simulink library "simulink"  (R2016b)
settings: Solver=ode45  StartTime=0.0  StopTime=10.0  RelTol=1e-3
PostLoadFcn:
  | setsysloc_simulink(bdroot)
undefined symbols (not defined in the file): DiscIntNeverNeededParam, docblock, getdatatypespecs, NumBits1, NumBits2, sfunxy, sigbuilder_block, slcm, SlDemoSign, Slope1, Slope2
libraries: simulink x37, sl_helperblocks x2, eml_lib x1
(part 6 of 6)

== system simulink/Sources/Chirp Signal ==
  note: freqSlope = deltaFreq/targetTime;
      | instantaneousFreq(t) = freqSlope*t + initialFreq;
      | intantaneousPhase(t) = integral(instFreq) = ...
      |       0.5*freqSlope*t^2 + initialFreq*t;
      | outputSignal(t) = sin(instantaneousPhase(t));
  Clock1 : Clock
      settings: DisableCoverage=on
  Gain : Gain  DisableCoverage=on  Gain=0.5  OutDataTypeStr=Inherit: Same as input  ParamDataTypeStr=Inherit: Same as input
  Output : Trigonometry
  Product : Product  DisableCoverage=on  Inputs=*/  SaturateOnIntegerOverflow=on  InputSameDT=on  OutDataTypeStr=Inherit: Same as first input
  Product1 : Product  DisableCoverage=on  SaturateOnIntegerOverflow=on  InputSameDT=on  OutDataTypeStr=Inherit: Same as first input
  Product2 : Product  DisableCoverage=on  SaturateOnIntegerOverflow=on  InputSameDT=on  OutDataTypeStr=Inherit: Same as first input
  Sum : Sum  DisableCoverage=on  Inputs=|++  SaturateOnIntegerOverflow=on  InputSameDT=on  OutDataTypeStr=Inherit: Same as first input
  deltaFreq : Constant  DisableCoverage=on  Value=2*pi*(f2-f1)
  initialFreq : Constant  DisableCoverage=on  Value=2*pi*f1
  targetTime : Constant  DisableCoverage=on  Value=T
  y : Outport
  wires:
  deltaFreq/1 -> Product/1
  targetTime/1 -> Product/2
  Product/1 -> Gain/1
  Clock1/1 -> Product1/1, Product2/1
  Gain/1 -> Product1/2
  Product1/1 -> Sum/1
  initialFreq/1 -> Sum/2
  Sum/1 -> Product2/2
  Product2/1 -> Output/1
  Output/1 -> y/1

== system simulink/Sources/Counter Free-Running ==
  FixPt Data Type Propagation : simulink/Signal Attributes/Data Type Propagation  PropDataTypeMode=Specify via dialog  PropDataType=uint(NumBits)  IfRefDouble=double  IfRefSingle=single  IsSigned=IsSigned1 or IsSigned2  NumBitsBase=max([NumBits1 NumBits2])  NumBitsMult=1  NumBitsAdd=0  NumBitsAllowFinal=1:128  PropScalingMode=Specify via dialog  PropScaling=1  ValuesUsedBestPrec=[5 -7]  SlopeBase=min([Slope1 Slope2])  SlopeMult=1  SlopeAdd=0  BiasBase=Bias1  BiasMult=1  BiasAdd=0
  Force to be scalar : SignalSpecification  DisableCoverage=on  Dimensions=1
  Increment Real World : simulink/Additional Math & Discrete/Additional Math: Increment - Decrement/Increment Real World  DisableCoverage=on
  Output : UnitDelay  InitialCondition=0.0  SampleTime=tsamp
  Wrap To Zero : simulink/Discontinuities/Wrap To Zero  DisableCoverage=on  Threshold=(2^(NumBits))-1
  y : Outport
  wires:
  Force to be scalar/1 -> Increment Real World/1
  Wrap To Zero/1 -> Output/1, FixPt Data Type Propagation/1, FixPt Data Type Propagation/3, FixPt Data Type Propagation/2
  Increment Real World/1 -> Wrap To Zero/1
  Output/1 -> Force to be scalar/1, y/1

== system simulink/Sources/Counter Limited ==
  Data Type Propagation : simulink/Signal Attributes/Data Type Propagation  PropDataTypeMode=Specify via dialog  PropDataType=uint(nbits)  IfRefDouble=double  IfRefSingle=single  IsSigned=IsSigned1 or IsSigned2  NumBitsBase=max([NumBits1 NumBits2])  NumBitsMult=1  NumBitsAdd=0  NumBitsAllowFinal=1:128  PropScalingMode=Specify via dialog  PropScaling=1  ValuesUsedBestPrec=[5 -7]  SlopeBase=min([Slope1 Slope2])  SlopeMult=1  SlopeAdd=0  BiasBase=Bias1  BiasMult=1  BiasAdd=0
  Force to be scalar : SignalSpecification  DisableCoverage=on  Dimensions=1
  Increment Real World : simulink/Additional Math & Discrete/Additional Math: Increment - Decrement/Increment Real World  DisableCoverage=on
  Output : UnitDelay  InitialCondition=0.0  SampleTime=tsamp
  Wrap To Zero : simulink/Discontinuities/Wrap To Zero  DisableCoverage=on  Threshold=uplimit
  y : Outport
  wires:
  Force to be scalar/1 -> Increment Real World/1
  Increment Real World/1 -> Wrap To Zero/1
  Output/1 -> Force to be scalar/1, y/1
  Wrap To Zero/1 -> Data Type Propagation/3, Data Type Propagation/2, Data Type Propagation/1, Output/1

== system simulink/Sources/Enumerated Constant ==
  Constant : Constant  DialogController=Simulink.DDGSource  Value=SlDemoSign.Positive  OutDataTypeStr=Enum: SlDemoSign  LockScale=on
  Out : Outport
  wires:
  Constant/1 -> Out/1

== system simulink/Sources/Ramp ==
  Clock : Clock
      settings: DisableCoverage=on
  Constant : Constant  DisableCoverage=on  Value=start  OutDataTypeStr=Inherit: Inherit via back propagation
  Constant1 : Constant  DisableCoverage=on  Value=X0  OutDataTypeStr=Inherit: Inherit via back propagation
  Output : Sum  Inputs=|++  SaturateOnIntegerOverflow=on  InputSameDT=on  OutDataTypeStr=Inherit: Same as first input
  Product : Product  DisableCoverage=on  SaturateOnIntegerOverflow=on  InputSameDT=on  OutDataTypeStr=Inherit: Same as first input
  Step : Step  DisableCoverage=on  Time=start  After=slope  SampleTime=0
  Sum : Sum  DisableCoverage=on  Inputs=|+-  SaturateOnIntegerOverflow=on  InputSameDT=on  OutDataTypeStr=Inherit: Same as first input
  Out1 : Outport
  wires:
  Step/1 -> Product/1
  Product/1 -> Output/1
  Constant1/1 -> Output/2
  Output/1 -> Out1/1
  Sum/1 -> Product/2
  Constant/1 -> Sum/2
  Clock/1 -> Sum/1

== system simulink/Sources/Repeating Sequence ==
  Clock : Clock
      settings: DisableCoverage=on
  Constant : Constant  DisableCoverage=on  Value=period
  Look-Up Table1 : Lookup_n-D  DisableCoverage=on  NumberOfTableDimensions=1  BreakpointsForDimension1=rep_seq_t - min(rep_seq_t)  BreakpointsForDimension3=[5, 7]  Table=rep_seq_y  InternalRulePriority=Speed  SaturateOnIntegerOverflow=on  InputSameDT=on
  Math Function : Math  DisableCoverage=on  Operator=rem  SaturateOnIntegerOverflow=on
  Output : SignalConversion  OverrideOpt=off
  Sum : Sum  DisableCoverage=on  Inputs=+-  SaturateOnIntegerOverflow=on  InputSameDT=on  OutDataTypeStr=Inherit: Same as first input
  startTime : S-Function  DisableCoverage=on  FunctionName=sfun_tstart  SFunctionDeploymentMode=off  EnableBusSupport=off
  Out1 : Outport
  wires:
  Math Function/1 -> Look-Up Table1/1
  Sum/1 -> Math Function/1
  Clock/1 -> Sum/1
  startTime/1 -> Sum/2
  Look-Up Table1/1 -> Output/1
  Output/1 -> Out1/1
  Constant/1 -> Math Function/2

== system simulink/Sources/Repeating Sequence Interpolated ==
  Data Type Propagation : simulink/Signal Attributes/Data Type Propagation  PropDataType=fixdt(1, 16)  IfRefDouble=double  IfRefSingle=single  IsSigned=IsSigned2  NumBitsBase=NumBits2  NumBitsMult=1  NumBitsAdd=0  NumBitsAllowFinal=1:128  PropScaling=2^-10  ValuesUsedBestPrec=[5 -7]  SlopeBase=Slope2  SlopeMult=1  SlopeAdd=0  BiasBase=Bias2  BiasMult=1  BiasAdd=0
  Data Type Conversion : DataTypeConversion  DisableCoverage=on
  Force to be scalar : SignalSpecification  DisableCoverage=on  Dimensions=1
  LimitedCounter : simulink/Sources/Counter Limited  uplimit=nn  tsamp=tsamp
  Lookup : Lookup_n-D  DisableCoverage=on  NumberOfTableDimensions=1  BreakpointsForDimension1=TimeValues  BreakpointsForDimension3=[5, 7]  Table=OutValues  ExtrapMethod=Clip  OutMin=OutMin  OutMax=OutMax  OutDataTypeStr=OutDataTypeStr  InputSameDT=on
  Output : SignalConversion  OverrideOpt=off
  Sample Time Math : SampleTimeMath  DisableCoverage=on  TsampMathOp=*  TsampMathImp=Offline Scaling Adjustment
  y : Outport  OutMin=OutMin  OutMax=OutMax
  wires:
  Output/1 -> y/1
  Lookup/1 -> Output/1, Data Type Propagation/1
  Force to be scalar/1 -> Data Type Conversion/1, Data Type Propagation/2
  LimitedCounter/1 -> Force to be scalar/1
  Sample Time Math/1 -> Lookup/1
  Data Type Conversion/1 -> Sample Time Math/1, Data Type Propagation/3

== system simulink/Sources/Repeating Sequence Stair ==
  Force to be scalar : SignalSpecification  DisableCoverage=on  Dimensions=1
  LimitedCounter : simulink/Sources/Counter Limited  uplimit=nn  tsamp=tsamp
  Out : SignalConversion  OverrideOpt=off
  Output : MultiPortSwitch  DisableCoverage=on  DataPortOrder=Zero-based contiguous  Inputs=1  zeroidx=on  OutMin=OutMin  OutMax=OutMax  SampleTime=tsamp
  Vector : Constant  DisableCoverage=on  Value=OutValues  OutMin=OutMin  OutMax=OutMax  OutDataTypeStr=OutDataTypeStr
  y : Outport  OutMin=OutMin  OutMax=OutMax
  wires:
  Force to be scalar/1 -> Output/1
  Vector/1 -> Output/2
  LimitedCounter/1 -> Force to be scalar/1
  Output/1 -> Out/1
  Out/1 -> y/1

== system simulink/Sources/Signal Builder ==
  Demux : Demux  Tag=STV Demux  Outputs=1
  FromWs : FromWorkspace  Tag=STV FromWs  VariableName=tuvar  SampleTime=0
      SigBuilderData=|
      | common.afterFinalStr = 'Extrapolate'
      | common.sampleTime = 0
      | dataSet.timeRange = [0 10]
      | dataSet.name = 'Group 1'
      | sbobj.Groups.Name = 'Group 1'
      | sbobj.Groups.Signals.Name = 'Signal 1'
      | sbobj.Groups.Signals.XData = [0 4 4 6 6 10]
      | sbobj.Groups.Signals.YData = [0 0 1 1 0 0]
  Signal 1 : Outport  Tag=STV Outport
  wires:
  FromWs/1 -> Demux/1
  Demux/1 -> Signal 1/1

== system simulink/Sources/Waveform Generator ==
  Converter : DataTypeConversion  OutMin=OutMin  OutMax=OutMax  OutDataTypeStr=double
  MultiportSwitch : MultiPortSwitch  Inputs=1
  MultiportSwitch_e3df3653d217406 : Ground  DisableCoverage=on
  Switch : Constant  DisableCoverage=on  Value=SelectedSignal
  Out1 : Outport
  wires:
  Switch/1 -> MultiportSwitch/1
  Converter/1 -> Out1/1
  MultiportSwitch/1 -> Converter/1
  MultiportSwitch_e3df3653d217406/1 -> MultiportSwitch/2

== system simulink/User-Defined Functions/Initialize Function ==
  Constant : Constant  DisableCoverage=on  Value=0
  Event Listener : EventListener  EventType=Initialize  EventName=reset
  State Writer : StateWriter
  wires:
  Constant/1 -> State Writer/1

== system simulink/User-Defined Functions/S-Function Examples ==
  Gain : Gain  SaturateOnIntegerOverflow=on  OutDataTypeStr=Inherit: Same as input  ParamDataTypeStr=Inherit: Same as input

== system simulink/User-Defined Functions/Simulink Function ==
  f : TriggerPort  TriggerType=function-call  IsSimulinkFunction=on  FunctionName=f  VariantControl=Variant
  u : ArgIn  DisableCoverage=on  ArgumentName=u
  y : ArgOut  DisableCoverage=on  ArgumentName=y
  wires:
  u/1 -> y/1

== system simulink/User-Defined Functions/Terminate Function ==
  Event Listener : EventListener  EventType=Terminate  EventName=reset
  State Reader : StateReader
  Terminator : Terminator
  wires:
  State Reader/1 -> Terminator/1

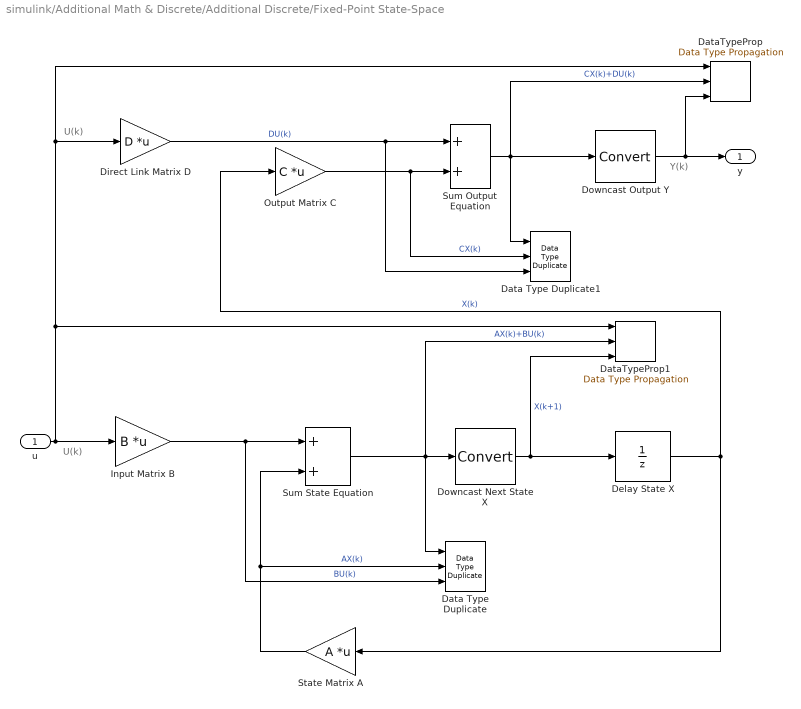
== system simulink/Additional Math & Discrete/Additional Discrete/Fixed-Point State-Space ==
  note: U(k)
  note: U(k)
  note: Y(k)
  u : Inport
  Data Type Duplicate : DataTypeDuplicate  DisableCoverage=on  NumInputPorts=3
  Data Type Duplicate1 : DataTypeDuplicate  DisableCoverage=on  NumInputPorts=3
  DataTypeProp : simulink/Signal Attributes/Data Type Propagation  PropDataType=fixdt(1, 16)  IfRefDouble=double  IfRefSingle=single  IsSigned=IsSigned1 or IsSigned2  NumBitsBase=NumBits1  NumBitsMult=1  NumBitsAdd=0  NumBitsAllowFinal=1:128  PropScaling=2^-10  ValuesUsedBestPrec=[5 -7]  SlopeBase=PosRange2  SlopeMult=1  SlopeAdd=0  BiasBase=Bias2  BiasMult=1  BiasAdd=0
  DataTypeProp1 : simulink/Signal Attributes/Data Type Propagation  PropDataType=fixdt(1, 16)  IfRefDouble=double  IfRefSingle=single  IsSigned=IsSigned1 or IsSigned2  NumBitsBase=NumBits1  NumBitsMult=1  NumBitsAdd=0  NumBitsAllowFinal=1:128  PropScaling=2^-10  ValuesUsedBestPrec=[5 -7]  SlopeBase=PosRange2  SlopeMult=1  SlopeAdd=0  BiasBase=Bias2  BiasMult=1  BiasAdd=0
  Delay State X : UnitDelay  Description=Store in Global RAM  DisableCoverage=on  InitialCondition=X0  SampleTime=-1
      settings: AttributesFormatString=%<Description>
  Direct Link Matrix D : Gain  Description=Multiply in CPU  DisableCoverage=on  Gain=D  Multiplication=Matrix(K*u) (u vector)  OutDataTypeStr=Inherit: Inherit via back propagation
      settings: AttributesFormatString=%<Description>
  Downcast Next State X : DataTypeConversion  Description=|  DisableCoverage=on
      | Reduce from CPU Size
      |  to Global RAM Size
      settings: AttributesFormatString=%<Description>
  Downcast Output Y : DataTypeConversion  Description=|
      | Reduce from CPU Size
      |  to Global RAM Size
      settings: AttributesFormatString=%<Description>
  Input Matrix B : Gain  Description=Multiply in CPU  DisableCoverage=on  Gain=B  Multiplication=Matrix(K*u) (u vector)  OutDataTypeStr=Inherit: Inherit via back propagation
      settings: AttributesFormatString=%<Description>
  Output Matrix C : Gain  Description=Multiply in CPU  DisableCoverage=on  Gain=C  Multiplication=Matrix(K*u) (u vector)  OutDataTypeStr=Inherit: Inherit via back propagation
      settings: AttributesFormatString=%<Description>
  State Matrix A : Gain  Description=Multiply in CPU  DisableCoverage=on  Gain=A  Multiplication=Matrix(K*u) (u vector)  OutDataTypeStr=Inherit: Inherit via back propagation
      settings: AttributesFormatString=%<Description>
  Sum Output Equation : Sum  Description=Add in CPU  DisableCoverage=on  OutDataTypeStr=slDataTypeAndScale(('InternalDataType'),('OutputEqScaling'))
      settings: AttributesFormatString=%<Description>
  Sum State Equation : Sum  Description=Add in CPU  DisableCoverage=on  OutDataTypeStr=slDataTypeAndScale(('InternalDataType'),('StateEqScaling'))
      settings: AttributesFormatString=%<Description>
  y : Outport  InitialOutput=0
  wires:
  Direct Link Matrix D/1 -> Data Type Duplicate1/3, Sum Output Equation/1  "DU(k)"
  Output Matrix C/1 -> Data Type Duplicate1/2, Sum Output Equation/2  "CX(k)"
  Sum Output Equation/1 -> DataTypeProp/2, Data Type Duplicate1/1, Downcast Output Y/1  "CX(k)+DU(k)"
  Downcast Output Y/1 -> DataTypeProp/3, y/1
  Delay State X/1 -> Output Matrix C/1, State Matrix A/1  "X(k)"
  Downcast Next State X/1 -> DataTypeProp1/3, Delay State X/1  "X(k+1)"
  Sum State Equation/1 -> DataTypeProp1/2, Data Type Duplicate/1, Downcast Next State X/1  "AX(k)+BU(k)"
  Input Matrix B/1 -> Data Type Duplicate/3, Sum State Equation/1  "BU(k)"
  u/1 -> DataTypeProp1/1, DataTypeProp/1, Direct Link Matrix D/1, Input Matrix B/1
  State Matrix A/1 -> Data Type Duplicate/2, Sum State Equation/2  "AX(k)"

== system simulink/Additional Math & Discrete/Additional Discrete/Transfer Fcn Direct Form II ==
  u : Inport
  DataTypeProp : simulink/Signal Attributes/Data Type Propagation  PropDataType=fixdt(1, 16)  IfRefDouble=double  IfRefSingle=single  IsSigned=IsSigned1 or IsSigned2  NumBitsBase=max([NumBits1 NumBits2])  NumBitsMult=1  NumBitsAdd=0  NumBitsAllowFinal=1:128  PropScaling=2^-10  ValuesUsedBestPrec=[5 -7]  SlopeBase=min([Slope1 Slope2])  SlopeMult=OutputSlopeMult  SlopeAdd=0  BiasBase=Bias1  BiasMult=0  BiasAdd=0
  DataTypeProp1 : simulink/Signal Attributes/Data Type Propagation  PropDataType=fixdt(1, 16)  IfRefDouble=double  IfRefSingle=single  IsSigned=IsSigned1 or IsSigned2  NumBitsBase=max([NumBits1 NumBits2])  NumBitsMult=1  NumBitsAdd=0  NumBitsAllowFinal=1:128  PropScaling=2^-10  ValuesUsedBestPrec=[5 -7]  SlopeBase=min([Slope1 Slope2])  SlopeMult=OutputSlopeMult2  SlopeAdd=0  BiasBase=Bias1  BiasMult=0  BiasAdd=0
  DenCoef : Gain  DisableCoverage=on  Gain=DenCoefVec  Multiplication=Matrix(K*u) (u vector)
      settings: AttributesFormatString=|
      | Data Type and Scaling Inherited
      | with goal of NO Quantization Noise
      | Possible Overflow or Saturation
  Downcast : DataTypeConversion  Description=|  LockScale=on
      | Reduce from CPU Size
      |  to Global RAM Size
      settings: AttributesFormatString=%<Description>
  Downcast1 : DataTypeConversion  Description=|  DisableCoverage=on  LockScale=on
      | Reduce from CPU Size
      |  to Global RAM Size
      settings: AttributesFormatString=%<Description>
  Mux : Mux  Inputs=2
  NumCoef : Gain  DisableCoverage=on  Gain=NumCoefVec  Multiplication=Matrix(K*u) (u vector)
      settings: AttributesFormatString=|
      | Data Type and Scaling Inherited
      | with goal of NO Quantization Noise
      | Possible Overflow or Saturation
  Sum : Sum  Tag=S16 2^-10  DisableCoverage=on  Inputs=+-  LockScale=on
      settings: AttributesFormatString=|
      | Data Type and Scaling Inherited
      | with goal of NO Quantization Noise
      | Possible Overflow or Saturation
  Tapped Delay : simulink/Discrete/Tapped Delay  vinit=vinit  samptime=-1  NumDelays=-1  DelayOrder=Newest  includeCurrent=off
      settings: AttributesFormatString=|
      | Number of Taps
      | Inherited via Back Propagation
  y : Outport
  wires:
  Sum/1 -> Downcast1/1
  DenCoef/1 -> Sum/2
  u/1 -> DataTypeProp1/1, DataTypeProp1/2, DataTypeProp/2, DataTypeProp/1, Sum/1
  NumCoef/1 -> Downcast/1
  Tapped Delay/1 -> DenCoef/1, Mux/2
  Downcast1/1 -> DataTypeProp1/3, Mux/1, Tapped Delay/1
  Mux/1 -> NumCoef/1
  Downcast/1 -> y/1, DataTypeProp/3

== system simulink/Additional Math & Discrete/Additional Discrete/Transfer Fcn Direct Form II Time Varying ==
  u : Inport
  Num : Inport  Port=2
  Den No Lead : Inport  Port=3
  DataTypeProp : simulink/Signal Attributes/Data Type Propagation  PropDataType=fixdt(1, 16)  IfRefDouble=double  IfRefSingle=single  IsSigned=IsSigned1  NumBitsBase=NumBits1  NumBitsMult=1  NumBitsAdd=0  NumBitsAllowFinal=1:128  PropScaling=2^-10  ValuesUsedBestPrec=[5 -7]  SlopeBase=Slope1  SlopeMult=1  SlopeAdd=0  BiasBase=Bias1  BiasMult=1  BiasAdd=0
  DataTypeProp1 : simulink/Signal Attributes/Data Type Propagation  PropDataType=fixdt(1, 16)  IfRefDouble=double  IfRefSingle=single  IsSigned=IsSigned1  NumBitsBase=NumBits1  NumBitsMult=1  NumBitsAdd=0  NumBitsAllowFinal=1:128  PropScaling=2^-10  ValuesUsedBestPrec=[5 -7]  SlopeBase=Slope1  SlopeMult=2  SlopeAdd=0  BiasBase=Bias1  BiasMult=1  BiasAdd=0
  Dot1 : DotProduct  DisableCoverage=on  OutDataTypeStr=Inherit: Inherit via internal rule
      settings: AttributesFormatString=|
      | Data Type and Scaling Inherited
      | with goal of NO Quantization Noise
      | Possible Overflow or Saturation
  Dot2 : DotProduct  DisableCoverage=on  OutDataTypeStr=Inherit: Inherit via internal rule
      settings: AttributesFormatString=|
      | Data Type and Scaling Inherited
      | with goal of NO Quantization Noise
      | Possible Overflow or Saturation
  Downcast : DataTypeConversion  Description=|  LockScale=on
      | Reduce from CPU Size
      |  to Global RAM Size
      settings: AttributesFormatString=%<Description>
  Downcast1 : DataTypeConversion  Description=|  DisableCoverage=on  LockScale=on
      | Reduce from CPU Size
      |  to Global RAM Size
      settings: AttributesFormatString=%<Description>
  Mux : Mux  Inputs=2
  Sum : Sum  Tag=S16 2^-10  DisableCoverage=on  Inputs=+-  LockScale=on
      settings: AttributesFormatString=|
      | Data Type and Scaling Inherited
      | with goal of NO Quantization Noise
      | Possible Overflow or Saturation
  Tapped Delay : simulink/Discrete/Tapped Delay  vinit=vinit  samptime=-1  NumDelays=-1  DelayOrder=Newest  includeCurrent=off
      settings: AttributesFormatString=|
      | Number of Taps
      | Inherited via Back Propagation
  y : Outport
  wires:
  Den No Lead/1 -> Dot1/2
  Num/1 -> Dot2/2
  Downcast/1 -> DataTypeProp/3, y/1
  Mux/1 -> Dot2/1
  Downcast1/1 -> DataTypeProp1/3, Tapped Delay/1, Mux/1
  Tapped Delay/1 -> Dot1/1, Mux/2
  Dot2/1 -> Downcast/1
  u/1 -> Sum/1, DataTypeProp1/2, DataTypeProp1/1, DataTypeProp/2, DataTypeProp/1
  Dot1/1 -> Sum/2
  Sum/1 -> Downcast1/1

== system simulink/Additional Math & Discrete/Additional Math: Increment - Decrement/Decrement Real World ==
  u : Inport
  FixPt Constant : Constant  DisableCoverage=on  OutDataTypeStr=Inherit: Inherit via back propagation
  FixPt Data Type Duplicate : DataTypeDuplicate  DisableCoverage=on  NumInputPorts=3
  FixPt Sum1 : Sum  Inputs=+-  OutDataTypeStr=Inherit: Inherit via back propagation  InputSameDT=on  LockScale=on
  y : Outport
  wires:
  FixPt Sum1/1 -> y/1, FixPt Data Type Duplicate/1
  FixPt Constant/1 -> FixPt Sum1/2, FixPt Data Type Duplicate/3
  u/1 -> FixPt Sum1/1, FixPt Data Type Duplicate/2

== system simulink/Additional Math & Discrete/Additional Math: Increment - Decrement/Decrement Stored Integer ==
  u : Inport
  FixPt Constant : Constant  DisableCoverage=on  OutDataTypeStr=Inherit: Inherit via back propagation
  FixPt Data Type Duplicate : DataTypeDuplicate  DisableCoverage=on  NumInputPorts=3
  FixPt Data Type Propagation : simulink/Signal Attributes/Data Type Propagation  PropDataType=fixdt(1, 16)  IfRefDouble=double  IfRefSingle=single  IsSigned=IsSigned1  NumBitsBase=NumBits1  NumBitsMult=1  NumBitsAdd=0  NumBitsAllowFinal=1:128  PropScaling=2^-10  ValuesUsedBestPrec=[5 -7]  SlopeBase=Slope1  SlopeMult=0  SlopeAdd=1  BiasBase=Bias1  BiasMult=0  BiasAdd=0
  FixPt Gateway In : DataTypeConversion  DisableCoverage=on  ConvertRealWorld=Stored Integer (SI)
  FixPt Sum1 : Sum  Inputs=+-  OutDataTypeStr=Inherit: Inherit via back propagation  InputSameDT=on  LockScale=on
  y : Outport
  wires:
  u/1 -> FixPt Data Type Duplicate/2, FixPt Sum1/1
  FixPt Constant/1 -> FixPt Gateway In/1, FixPt Data Type Propagation/3
  FixPt Sum1/1 -> FixPt Data Type Duplicate/1, y/1
  FixPt Gateway In/1 -> FixPt Data Type Duplicate/3, FixPt Sum1/2, FixPt Data Type Propagation/1, FixPt Data Type Propagation/2

== system simulink/Additional Math & Discrete/Additional Math: Increment - Decrement/Decrement To Zero ==
  u : Inport
  FixPt Constant : Constant  DisableCoverage=on  OutDataTypeStr=Inherit: Inherit via back propagation
  FixPt Data Type Duplicate : DataTypeDuplicate  DisableCoverage=on  NumInputPorts=5
  FixPt Relational Operator3 : RelationalOperator  DisableCoverage=on  Operator=>  OutDataTypeStr=boolean  ZeroCross=off  RndMeth=Nearest
  FixPt Sum1 : Sum  DisableCoverage=on  Inputs=+-  OutDataTypeStr=Inherit: Inherit via back propagation  LockScale=on
  FixPt Switch4 : Switch  Criteria=u2 ~= 0  Threshold=1  OutDataTypeStr=Inherit: Inherit via back propagation  ZeroCross=off
  Ground1 : Ground  DisableCoverage=on
  y : Outport
  wires:
  FixPt Switch4/1 -> FixPt Data Type Duplicate/1, y/1
  Ground1/1 -> FixPt Data Type Duplicate/2, FixPt Switch4/3
  FixPt Relational Operator3/1 -> FixPt Switch4/2
  u/1 -> FixPt Relational Operator3/1, FixPt Data Type Duplicate/4, FixPt Sum1/1
  FixPt Constant/1 -> FixPt Relational Operator3/2, FixPt Data Type Duplicate/5, FixPt Sum1/2
  FixPt Sum1/1 -> FixPt Switch4/1, FixPt Data Type Duplicate/3

== system simulink/Additional Math & Discrete/Additional Math: Increment - Decrement/Decrement Time To Zero ==
  u : Inport
  FixPt Data Type Duplicate : DataTypeDuplicate  DisableCoverage=on  NumInputPorts=5
  FixPt Relational Operator3 : RelationalOperator  DisableCoverage=on  Operator=>  OutDataTypeStr=boolean  ZeroCross=off  RndMeth=Nearest
  FixPt Sample Time Math : SampleTimeMath  DisableCoverage=on  TsampMathOp=Ts Only  OutDataTypeStr=Inherit: Inherit via back propagation
  FixPt Sum1 : Sum  DisableCoverage=on  Inputs=+-  OutDataTypeStr=Inherit: Inherit via back propagation  LockScale=on
  FixPt Switch4 : Switch  Criteria=u2 ~= 0  Threshold=1  OutDataTypeStr=Inherit: Inherit via back propagation  ZeroCross=off
  Ground1 : Ground  DisableCoverage=on
  y : Outport
  wires:
  FixPt Switch4/1 -> FixPt Data Type Duplicate/1, y/1
  Ground1/1 -> FixPt Data Type Duplicate/2, FixPt Switch4/3
  FixPt Relational Operator3/1 -> FixPt Switch4/2
  u/1 -> FixPt Relational Operator3/1, FixPt Data Type Duplicate/4, FixPt Sum1/1, FixPt Sample Time Math/1
  FixPt Sample Time Math/1 -> FixPt Relational Operator3/2, FixPt Data Type Duplicate/5, FixPt Sum1/2
  FixPt Sum1/1 -> FixPt Switch4/1, FixPt Data Type Duplicate/3

== system simulink/Additional Math & Discrete/Additional Math: Increment - Decrement/Increment Real World ==
  u : Inport
  FixPt Constant : Constant  DisableCoverage=on  OutDataTypeStr=Inherit: Inherit via back propagation
  FixPt Data Type Duplicate : DataTypeDuplicate  DisableCoverage=on  NumInputPorts=3
  FixPt Sum1 : Sum  OutDataTypeStr=Inherit: Inherit via back propagation  InputSameDT=on  LockScale=on
  y : Outport
  wires:
  u/1 -> FixPt Data Type Duplicate/2, FixPt Sum1/1
  FixPt Constant/1 -> FixPt Data Type Duplicate/3, FixPt Sum1/2
  FixPt Sum1/1 -> FixPt Data Type Duplicate/1, y/1

== system simulink/Additional Math & Discrete/Additional Math: Increment - Decrement/Increment Stored Integer ==
  u : Inport
  FixPt Constant : Constant  DisableCoverage=on  OutDataTypeStr=Inherit: Inherit via back propagation
  FixPt Data Type Duplicate : DataTypeDuplicate  DisableCoverage=on  NumInputPorts=3
  FixPt Data Type Propagation : simulink/Signal Attributes/Data Type Propagation  PropDataType=fixdt(1, 16)  IfRefDouble=double  IfRefSingle=single  IsSigned=IsSigned1  NumBitsBase=NumBits1  NumBitsMult=1  NumBitsAdd=0  NumBitsAllowFinal=1:128  PropScaling=2^-10  ValuesUsedBestPrec=[5 -7]  SlopeBase=Slope1  SlopeMult=0  SlopeAdd=1  BiasBase=Bias1  BiasMult=0  BiasAdd=0
  FixPt Gateway In : DataTypeConversion  DisableCoverage=on  ConvertRealWorld=Stored Integer (SI)
  FixPt Sum1 : Sum  OutDataTypeStr=Inherit: Inherit via back propagation  InputSameDT=on  LockScale=on
  y : Outport
  wires:
  FixPt Gateway In/1 -> FixPt Data Type Propagation/2, FixPt Data Type Propagation/1, FixPt Sum1/2, FixPt Data Type Duplicate/3
  FixPt Sum1/1 -> y/1, FixPt Data Type Duplicate/1
  FixPt Constant/1 -> FixPt Data Type Propagation/3, FixPt Gateway In/1
  u/1 -> FixPt Sum1/1, FixPt Data Type Duplicate/2

== system simulink/Model Verification/Check Input Resolution/fixed ==
  u : Inport
  resolution : Inport  Port=2
  fold : Logic  DisableCoverage=on  Operator=OR  Inputs=1
  relop : RelationalOperator  DisableCoverage=on  Operator===  RndMeth=Nearest  InputSameDT=on
  out : Outport
  wires:
  u/1 -> relop/1
  resolution/1 -> relop/2
  relop/1 -> fold/1
  fold/1 -> out/1

== system simulink/Model Verification/Check Input Resolution/steps ==
  u : Inport
  resolution : Inport  Port=2
  relop : RelationalOperator  DisableCoverage=on  Operator=<=  RndMeth=Nearest  InputSameDT=on
  rem : Math  DisableCoverage=on  Operator=mod  SaturateOnIntegerOverflow=on
  tol : Constant  DisableCoverage=on  Value=10e-3
  out : Outport
  wires:
  u/1 -> rem/1
  resolution/1 -> rem/2
  rem/1 -> relop/1
  tol/1 -> relop/2
  relop/1 -> out/1

== system simulink/Model-Wide Utilities/Block Support Table/EmptySubsystem ==

== system simulink/Model-Wide Utilities/DocBlock/EmptySubsystem ==

== system simulink/Model-Wide Utilities/Model Info/EmptySubsystem ==

== system simulink/Model-Wide Utilities/Timed-Based Linearization/Triggered Linearization ==
  Trigger : TriggerPort  VariantControl=Variant
  MATLAB S-Function : M-S-Function  DisableCoverage=on  FunctionName=sfunlin  Parameters=name_,SampleTime
